simulink model "qpsk_vs_msk_live"  (Simulink 7.7)
settings: Solver=ode45  StartTime=0.0  StopTime=1e4  FixedStep=1  RelTol=1e-3
values from neighbouring files (symbols this model uses):
  Fs = 2000    [DAC_fft.m]    (also in FFT_iFFT.m = 5000; InterpolateSignalVector.m = 600; RCpulsePSD.m = 200000; RaisedCos_shaping_example.m = 8000)
undefined symbols (not defined in the file or in its folder): figposition, get, sided, Two, upsamp
libraries: commsink2 x11, simulink x7, commchan3 x4, commdigbbndpm3 x3, commfilt2 x3, dspsnks4 x3, commrandsrc2 x2, commblksprivate x1, commdigbbndcpm2 x1
Description:
  | Filtered QPSK vs. MSK
  | 
  | This demo enables you to visually compare filtered quadrature phase shift keying (QPSK) and minimum shift keying (MSK) modulation schemes.
CloseFcn:
  | clear qpskSigsOut
settings Model: Creator=The MathWorks Inc.  LastModifiedBy=mainster  ExtModeAutoUpdateStatusClock=off
settings DataIOCC: LimitDataPoints=off  SaveOutput=off  SaveTime=off  SignalLoggingName=qpskSigsOut
settings OptimizationCC: InlineInvariantSignals=on  InitFltsAndDblsToZero=on  EfficientMapNaN2IntZero=off
settings DebuggingCC: SaveWithParameterizedLinksMsg=none  CheckExecutionContextPreStartOutputMsg=on  CheckExecutionContextRuntimeOutputMsg=on  SignalResolutionControl=TryResolveAllWithWarning  SolverPrmCheckMsg=none  InheritedTsInSrcMsg=none  MultiTaskDSMMsg=warning  MultiTaskCondExecSysMsg=none  SigSpecEnsureSampleTimeMsg=none  StrictBusMsg=None
settings HardwareCC: TargetUnknown=on
settings ModelReferenceCC: UpdateModelReferenceTargets=IfOutOfDate
settings RTWCC: IncludeERTFirstTime=on
settings GRTTargetCC: TargetFcnLib=ansi_tfl_tmw.mat

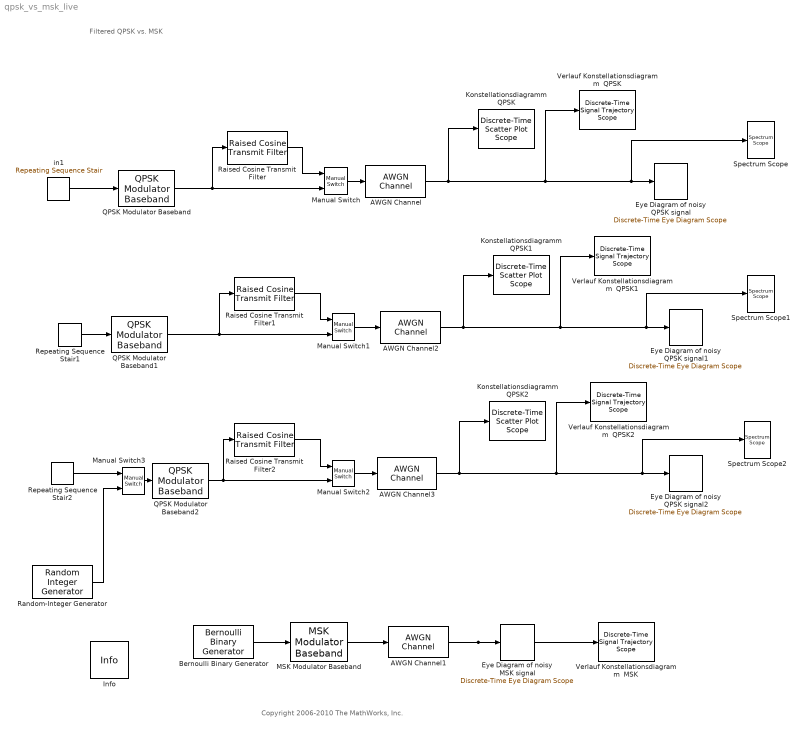
== system qpsk_vs_msk_live ==
  note: Filtered QPSK vs. MSK
  note: Copyright 2006-2010 The MathWorks, Inc.
  AWGN Channel : commchan3/AWGN Channel  SystemSampleTime=-1  InputProcessing=Columns as channels (frame based)  seed=1237  noiseMode="Signal to noise ratio  (SNR)"  EbNodB=10  EsNodB=10  SNRdB=25  bitsPerSym=1  Ps=1  Tsym=1  variance=1
  AWGN Channel1 : commchan3/AWGN Channel  SystemSampleTime=-1  InputProcessing=Columns as channels (frame based)  seed=1237  noiseMode="Signal to noise ratio  (SNR)"  EbNodB=10  EsNodB=10  SNRdB=30  bitsPerSym=1  Ps=1  Tsym=1  variance=1
  AWGN Channel2 : commchan3/AWGN Channel  SystemSampleTime=-1  InputProcessing=Columns as channels (frame based)  seed=1237  noiseMode="Signal to noise ratio  (SNR)"  EbNodB=10  EsNodB=10  SNRdB=25  bitsPerSym=1  Ps=1  Tsym=1  variance=1
  AWGN Channel3 : commchan3/AWGN Channel  SystemSampleTime=-1  InputProcessing=Columns as channels (frame based)  seed=1237  noiseMode="Signal to noise ratio  (SNR)"  EbNodB=10  EsNodB=10  SNRdB=25  bitsPerSym=1  Ps=1  Tsym=1  variance=1
  Bernoulli Binary Generator : commrandsrc2/Bernoulli Binary Generator  SystemSampleTime=-1  P=0.5  seed=61  Ts=0.5  frameBased=off  sampPerFrame=1  orient=off  outDataType=boolean
  Eye Diagram of noisy MSK signal : commsink2/Discrete-Time Eye Diagram Scope  Tag=EyeDiagram  SystemSampleTime=-1  sampPerSymb=8  offsetEye=4  symbPerTrace=4  numTraces=40  numNewFrames=10  LineStyles=-  LineColors=m  dupPoints=on  fading=on  render=on  AxisGrid=on  yMin=-1.5  yMax=1.5  inphaseLabel=In-phase Amplitude  quadratureLabel=Quadrature Amplitude  openScopeAtSimStart=off  dispDiagram=In-phase and Quadrature  FrameNumber=off  FigPos=figposition([1 5 30 65])  figTitle=Eye Diagram of Noisy MSK Signal  block_type_=eye  numLinesMax=8
  Eye Diagram of noisy QPSK signal : commsink2/Discrete-Time Eye Diagram Scope  Tag=EyeDiagram  SystemSampleTime=-1  sampPerSymb=lengthOfSymbol  offsetEye=0  symbPerTrace=2  numTraces=40  numNewFrames=10  LineStyles=-  LineColors=b  dupPoints=on  fading=on  render=on  AxisGrid=on  yMin=-1.5  yMax=1.5  inphaseLabel=In-phase Amplitude  quadratureLabel=Quadrature Amplitude  openScopeAtSimStart=off  dispDiagram=In-phase and Quadrature  FrameNumber=off  FigPos=figposition([66 5 30 65])  figTitle=Eye Diagram of Noisy QPSK Signal  block_type_=eye  numLinesMax=8
  Eye Diagram of noisy QPSK signal1 : commsink2/Discrete-Time Eye Diagram Scope  Tag=EyeDiagram  SystemSampleTime=-1  sampPerSymb=8  offsetEye=0  symbPerTrace=2  numTraces=40  numNewFrames=10  LineStyles=-  LineColors=b  dupPoints=on  fading=on  render=on  AxisGrid=on  yMin=-1.5  yMax=1.5  inphaseLabel=In-phase Amplitude  quadratureLabel=Quadrature Amplitude  openScopeAtSimStart=off  dispDiagram=In-phase and Quadrature  FrameNumber=off  FigPos=figposition([66 5 30 65])  figTitle=Eye Diagram of Noisy QPSK Signal  block_type_=eye  numLinesMax=8
  Eye Diagram of noisy QPSK signal2 : commsink2/Discrete-Time Eye Diagram Scope  Tag=EyeDiagram  SystemSampleTime=-1  sampPerSymb=8  offsetEye=0  symbPerTrace=2  numTraces=40  numNewFrames=10  LineStyles=-  LineColors=b  dupPoints=on  fading=on  render=on  AxisGrid=on  yMin=-1.5  yMax=1.5  inphaseLabel=In-phase Amplitude  quadratureLabel=Quadrature Amplitude  openScopeAtSimStart=off  dispDiagram=In-phase and Quadrature  FrameNumber=off  FigPos=figposition([66 5 30 65])  figTitle=Eye Diagram of Noisy QPSK Signal  block_type_=eye  numLinesMax=8
  Info : commblksprivate/Info  SystemSampleTime=-1
  Konstellationsdiagramm QPSK : commsink2/Discrete-Time Scatter Plot Scope  Tag=ScatterPlot  SystemSampleTime=-1  sampPerSymb=lengthOfSymbol  offsetEye=0  numTraces=150  numNewFrames=20  LineMarkers=.  LineColors=b  fading=on  render=on  AxisGrid=on  xMin=-1.3  xMax=1.315  yMin=-1.3  yMax=1.315  inphaseLabel=Amplitude Realteil  quadratureLabel=Amplitude Imaginaerteil  openScopeAtSimStart=on  FrameNumber=off  FigPos=get(0,'defaultfigureposition');  figTitle=Konstellationsdiagramm  numLinesMax=8  block_type_=scatter
  Konstellationsdiagramm QPSK1 : commsink2/Discrete-Time Scatter Plot Scope  Tag=ScatterPlot  SystemSampleTime=-1  sampPerSymb=lengthOfSymbol  offsetEye=0  numTraces=150  numNewFrames=20  LineMarkers=.  LineColors=b  fading=on  render=on  AxisGrid=on  xMin=-1.3  xMax=1.315  yMin=-1.3  yMax=1.315  inphaseLabel=Amplitude Realteil  quadratureLabel=Amplitude Imaginaerteil  openScopeAtSimStart=on  FrameNumber=off  FigPos=get(0,'defaultfigureposition');  figTitle=Konstellationsdiagramm  numLinesMax=8  block_type_=scatter
  Konstellationsdiagramm QPSK2 : commsink2/Discrete-Time Scatter Plot Scope  Tag=ScatterPlot  SystemSampleTime=-1  sampPerSymb=lengthOfSymbol  offsetEye=0  numTraces=150  numNewFrames=20  LineMarkers=.  LineColors=b  fading=on  render=on  AxisGrid=on  xMin=-1.3  xMax=1.315  yMin=-1.3  yMax=1.315  inphaseLabel=Amplitude Realteil  quadratureLabel=Amplitude Imaginaerteil  openScopeAtSimStart=on  FrameNumber=off  FigPos=get(0,'defaultfigureposition');  figTitle=Konstellationsdiagramm  numLinesMax=8  block_type_=scatter
  MSK Modulator Baseband : commdigbbndcpm2/MSK Modulator Baseband  SystemSampleTime=-1  inputType=Bit  phaseOffset=0  samplesPerSymbol=8  RateOptions=Allow multirate processing  outDataType=double
  Manual Switch : simulink/Signal Routing/Manual Switch  SystemSampleTime=-1  sw=1  action=0  varsize=off
  Manual Switch1 : simulink/Signal Routing/Manual Switch  SystemSampleTime=-1  sw=1  action=0  varsize=off
  Manual Switch2 : simulink/Signal Routing/Manual Switch  SystemSampleTime=-1  sw=1  action=0  varsize=off
  Manual Switch3 : simulink/Signal Routing/Manual Switch  SystemSampleTime=-1  sw=0  action=0  varsize=off
  QPSK Modulator Baseband : commdigbbndpm3/QPSK Modulator Baseband  SystemSampleTime=-1  InType=Integer  Enc=Gray  Ph=0  outDtype=double  outWordLen=16  outUDDataType=sfix(16)  outFracLenMode=Best precision  outFracLen=15
  QPSK Modulator Baseband1 : commdigbbndpm3/QPSK Modulator Baseband  SystemSampleTime=-1  InType=Integer  Enc=Gray  Ph=0  outDtype=double  outWordLen=16  outUDDataType=sfix(16)  outFracLenMode=Best precision  outFracLen=15
  QPSK Modulator Baseband2 : commdigbbndpm3/QPSK Modulator Baseband  SystemSampleTime=-1  InType=Integer  Enc=Gray  Ph=0  outDtype=double  outWordLen=16  outUDDataType=sfix(16)  outFracLenMode=Best precision  outFracLen=15
  Raised Cosine Transmit Filter : commfilt2/Raised Cosine Transmit Filter  SystemSampleTime=-1  filtType=Normal  D=1  R=0.3  sampMode=Mute  saveAsFlag=0  N=upsamp  framing=Allow multirate processing  checkGain=Normalized  filterGain=1  checkCoeff=off  variableName=rcTxFilt  launchFVT=off  roundingMode=Floor  overflowMode=off
  Raised Cosine Transmit Filter1 : commfilt2/Raised Cosine Transmit Filter  SystemSampleTime=-1  filtType=Normal  D=1  R=0.3  sampMode=Mute  saveAsFlag=0  N=upsamp  framing=Allow multirate processing  checkGain=Normalized  filterGain=1  checkCoeff=off  variableName=rcTxFilt1  launchFVT=off  roundingMode=Floor  overflowMode=off
  Raised Cosine Transmit Filter2 : commfilt2/Raised Cosine Transmit Filter  SystemSampleTime=-1  filtType=Normal  D=1  R=0.3  sampMode=Mute  saveAsFlag=0  N=upsamp  framing=Allow multirate processing  checkGain=Normalized  filterGain=1  checkCoeff=off  variableName=rcTxFilt2  launchFVT=off  roundingMode=Floor  overflowMode=off
  Random-Integer Generator : commrandsrc2/Random Integer Generator  SystemSampleTime=-1  mul=4  seed=[12345]  Ts=1  frameBased=off  sampPerFrame=50  orient=off  outDataType=int8
  Repeating Sequence Stair1 : simulink/Sources/Repeating Sequence Stair  SystemSampleTime=-1  OutValues=[0 1 2 3].'  tsamp=1  OutMin=[]  OutMax=[]  OutDataTypeStr=int8  OutputDataTypeScalingMode=int8  OutDataType=fixdt(0,8)  ConRadixGroup=Best Precision: Vector-wise  OutScaling=2^-12
  Repeating Sequence Stair2 : simulink/Sources/Repeating Sequence Stair  SystemSampleTime=-1  OutValues=[0 2 3 1].'  tsamp=1  OutMin=[]  OutMax=[]  OutDataTypeStr=int8  OutputDataTypeScalingMode=int8  OutDataType=fixdt(0,8)  ConRadixGroup=Best Precision: Vector-wise  OutScaling=2^-12
  Spectrum Scope : dspsnks4/Spectrum Scope  SystemSampleTime=-1  ScopeProperties=on  Domain=Frequency  HorizSpan=1  UseBuffer=on  BufferSize=128  Overlap=0  TreatMby1Signals=M channels  inpFftLenInherit=on  FFTlength=128  numAvg=2  DisplayProperties=off  AxisGrid=on  Memory=off  FrameNumber=on  AxisLegend=on  AxisZoom=off  OpenScopeAtSimStart=on  OpenScopeImmediately=off  FigPos=get(0,'defaultfigureposition')  AxisProperties=off  XUnits=Hertz  XRange=Two-sided ((-Fs/2...Fs/2])  XDisplay=0  InheritXIncr=on  XIncr=1.0  XLabel=Samples  XLimit=Auto  YUnits=dBm  XMax=1  XMin=0  YLabel=Magnitude-squared, dB  LineProperties=off  LineDisables=on | on  LineStyles=- | -  LineMarkers=. | .  LineColors=Red | Blue  wintypeSpecScope=Blackman  RsSpecScope=50  betaSpecScope=5  winsampSpecScope=Periodic  XAxisParamsVer=6.9  isFrameUpgraded=on
      settings: YMin=-10  YMax=10
  Spectrum Scope1 : dspsnks4/Spectrum Scope  SystemSampleTime=-1  ScopeProperties=on  Domain=Frequency  HorizSpan=1  UseBuffer=on  BufferSize=128  Overlap=0  TreatMby1Signals=M channels  inpFftLenInherit=on  FFTlength=128  numAvg=2  DisplayProperties=off  AxisGrid=on  Memory=off  FrameNumber=on  AxisLegend=on  AxisZoom=off  OpenScopeAtSimStart=on  OpenScopeImmediately=off  FigPos=get(0,'defaultfigureposition')  AxisProperties=off  XUnits=Hertz  XRange=Two-sided ((-Fs/2...Fs/2])  XDisplay=0  InheritXIncr=on  XIncr=1.0  XLabel=Samples  XLimit=Auto  YUnits=dBm  XMax=1  XMin=0  YLabel=Magnitude-squared, dB  LineProperties=off  LineDisables=on | on  LineStyles=- | -  LineMarkers=. | .  LineColors=Red | Blue  wintypeSpecScope=Blackman  RsSpecScope=50  betaSpecScope=5  winsampSpecScope=Periodic  XAxisParamsVer=6.9  isFrameUpgraded=on
      settings: YMin=-10  YMax=10
  Spectrum Scope2 : dspsnks4/Spectrum Scope  SystemSampleTime=-1  ScopeProperties=on  Domain=Frequency  HorizSpan=1  UseBuffer=on  BufferSize=128  Overlap=0  TreatMby1Signals=M channels  inpFftLenInherit=on  FFTlength=128  numAvg=2  DisplayProperties=off  AxisGrid=on  Memory=off  FrameNumber=on  AxisLegend=on  AxisZoom=off  OpenScopeAtSimStart=on  OpenScopeImmediately=off  FigPos=get(0,'defaultfigureposition')  AxisProperties=off  XUnits=Hertz  XRange=Two-sided ((-Fs/2...Fs/2])  XDisplay=0  InheritXIncr=on  XIncr=1.0  XLabel=Samples  XLimit=Auto  YUnits=dBm  XMax=1  XMin=0  YLabel=Magnitude-squared, dB  LineProperties=off  LineDisables=on | on  LineStyles=- | -  LineMarkers=. | .  LineColors=Red | Blue  wintypeSpecScope=Blackman  RsSpecScope=50  betaSpecScope=5  winsampSpecScope=Periodic  XAxisParamsVer=6.9  isFrameUpgraded=on
      settings: YMin=-10  YMax=10
  Verlauf Konstellationsdiagramm  MSK : commsink2/Discrete-Time Signal Trajectory Scope  Tag=SignalTrajectory  SystemSampleTime=-1  sampPerSymb=lengthOfSymbol  offsetEye=0  numTraces=40  numNewFrames=10  LineStyles=-  LineColors=b  fading=on  render=on  AxisGrid=on  xMin=-1.3  xMax=1.315  yMin=-1.3  yMax=1.315  inphaseLabel=Amplitude Realteil  quadratureLabel=Amplitude Imaginaerteil  openScopeAtSimStart=off  FrameNumber=on  FigPos=get(0,'defaultfigureposition');  figTitle=Verlauf Konstellationsdiagramm  numLinesMax=8  block_type_=xy
  Verlauf Konstellationsdiagramm  QPSK : commsink2/Discrete-Time Signal Trajectory Scope  Tag=SignalTrajectory  SystemSampleTime=-1  sampPerSymb=lengthOfSymbol  offsetEye=0  numTraces=40  numNewFrames=10  LineStyles=-  LineColors=b  fading=on  render=on  AxisGrid=on  xMin=-1.3  xMax=1.315  yMin=-1.3  yMax=1.315  inphaseLabel=Amplitude Realteil  quadratureLabel=Amplitude Imaginaerteil  openScopeAtSimStart=on  FrameNumber=on  FigPos=get(0,'defaultfigureposition');  figTitle=Verlauf Konstellationsdiagramm  numLinesMax=8  block_type_=xy
  Verlauf Konstellationsdiagramm  QPSK1 : commsink2/Discrete-Time Signal Trajectory Scope  Tag=SignalTrajectory  SystemSampleTime=-1  sampPerSymb=lengthOfSymbol  offsetEye=0  numTraces=40  numNewFrames=10  LineStyles=-  LineColors=b  fading=on  render=on  AxisGrid=on  xMin=-1.3  xMax=1.315  yMin=-1.3  yMax=1.315  inphaseLabel=Amplitude Realteil  quadratureLabel=Amplitude Imaginaerteil  openScopeAtSimStart=on  FrameNumber=on  FigPos=get(0,'defaultfigureposition');  figTitle=Verlauf Konstellationsdiagramm  numLinesMax=8  block_type_=xy
  Verlauf Konstellationsdiagramm  QPSK2 : commsink2/Discrete-Time Signal Trajectory Scope  Tag=SignalTrajectory  SystemSampleTime=-1  sampPerSymb=lengthOfSymbol  offsetEye=0  numTraces=40  numNewFrames=10  LineStyles=-  LineColors=b  fading=on  render=on  AxisGrid=on  xMin=-1.45121278222582  xMax=1.49463100350394  yMin=-1.48378526848284  yMax=1.46205851724693  inphaseLabel=Amplitude Realteil  quadratureLabel=Amplitude Imaginaerteil  openScopeAtSimStart=on  FrameNumber=on  FigPos=get(0,'defaultfigureposition');  figTitle=Verlauf Konstellationsdiagramm  numLinesMax=8  block_type_=xy
  in1 : simulink/Sources/Repeating Sequence Stair  SystemSampleTime=-1  OutValues=[0 1 2 3 2 1].'  tsamp=1  OutMin=[]  OutMax=[]  OutDataTypeStr=int8  OutputDataTypeScalingMode=int8  OutDataType=fixdt(0,8)  ConRadixGroup=Best Precision: Vector-wise  OutScaling=2^-12
  wires:
  Bernoulli Binary Generator/1 -> MSK Modulator Baseband/1
  MSK Modulator Baseband/1 -> AWGN Channel1/1
  AWGN Channel1/1 -> Eye Diagram of noisy MSK signal/1, Verlauf Konstellationsdiagramm  MSK/1
  QPSK Modulator Baseband/1 -> Manual Switch/2, Raised Cosine Transmit Filter/1
  AWGN Channel/1 -> Verlauf Konstellationsdiagramm  QPSK/1, Eye Diagram of noisy QPSK signal/1, Spectrum Scope/1, Konstellationsdiagramm QPSK/1
  in1/1 -> QPSK Modulator Baseband/1
  AWGN Channel2/1 -> Verlauf Konstellationsdiagramm  QPSK1/1, Eye Diagram of noisy QPSK signal1/1, Spectrum Scope1/1, Konstellationsdiagramm QPSK1/1
  Repeating Sequence Stair1/1 -> QPSK Modulator Baseband1/1
  AWGN Channel3/1 -> Verlauf Konstellationsdiagramm  QPSK2/1, Eye Diagram of noisy QPSK signal2/1, Spectrum Scope2/1, Konstellationsdiagramm QPSK2/1
  Raised Cosine Transmit Filter/1 -> Manual Switch/1
  Manual Switch/1 -> AWGN Channel/1
  QPSK Modulator Baseband1/1 -> Manual Switch1/2, Raised Cosine Transmit Filter1/1
  Raised Cosine Transmit Filter1/1 -> Manual Switch1/1
  Manual Switch1/1 -> AWGN Channel2/1
  Raised Cosine Transmit Filter2/1 -> Manual Switch2/1
  QPSK Modulator Baseband2/1 -> Manual Switch2/2, Raised Cosine Transmit Filter2/1
  Manual Switch2/1 -> AWGN Channel3/1
  Manual Switch3/1 -> QPSK Modulator Baseband2/1
  Random-Integer Generator/1 -> Manual Switch3/2
  Repeating Sequence Stair2/1 -> Manual Switch3/1
